simulink model "EMT_load"  (R2024a)
settings: Solver=ode1  StartTime=0.0  StopTime=simtime  FixedStep=Ts  RelTol=1e-3
values from neighbouring files (symbols this model uses):
  c0 = c0_hawk    (= 6.37282e-09)    [EMT_Phasor_parameters.m]
  c1 = c1_hawk    (= 8.76156e-09)    [EMT_Phasor_parameters.m]
  fg = 50    [EMT_Phasor_parameters.m]
  G1gen = 0.1245    [EMT_Phasor_parameters.m]
  G2gen = 0.30    (= 0.3)    [EMT_Phasor_parameters.m]
  G3gen = 0.20    (= 0.2)    [EMT_Phasor_parameters.m]
  G4sgen = 0.2078    [EMT_Phasor_parameters.m]
  G5gen = 0.20    (= 0.2)    [EMT_Phasor_parameters.m]
  G6gen = 0.2078    [EMT_Phasor_parameters.m]
  G6sgen = 0.20    (= 0.2)    [EMT_Phasor_parameters.m]
  G7gen = 0.518    [EMT_Phasor_parameters.m]
  Ihvpk = Ihv*sqrt(2)    [EMT_Phasor_parameters.m]
  l0 = l0_hawk    (= 0.00373)    [EMT_Phasor_parameters.m]
  l1 = l1_hawk    (= 0.00133)    [EMT_Phasor_parameters.m]
  L3dem = 0.10    (= 0.1)    [EMT_Phasor_parameters.m]
  L4dem = 0.30    (= 0.3)    [EMT_Phasor_parameters.m]
  L5dem = 0.35    [EMT_Phasor_parameters.m]
  L6dem = 0.15    [EMT_Phasor_parameters.m]
  L7dem = 0.10    (= 0.1)    [EMT_Phasor_parameters.m]
  Pr = Sr*PF    (= 550050000)    [EMT_Phasor_parameters.m]
  Qr = sqrt(Sr^2 - Pr^2)    [EMT_Phasor_parameters.m]
  r0 = r0_hawk    (= 0.44587)    [EMT_Phasor_parameters.m]
  r1 = r1_hawk    (= 0.12087)    [EMT_Phasor_parameters.m]
  Rtpu = Xtpu/40    (= 0.00375)    [EMT_Phasor_parameters.m]
  S1non = 400e6    (= 400000000)    [EMT_Phasor_parameters.m]
  S2non = 300e6    (= 300000000)    [EMT_Phasor_parameters.m]
  S3non = 200e6    (= 200000000)    [EMT_Phasor_parameters.m]
  S4snon = 200e6    (= 200000000)    [EMT_Phasor_parameters.m]
  S5non = 500e6    (= 500000000)    [EMT_Phasor_parameters.m]
  S6non = 400e6    (= 400000000)    [EMT_Phasor_parameters.m]
  S6snon = 200e6    (= 200000000)    [EMT_Phasor_parameters.m]
  S7non = 200e6    (= 200000000)    [EMT_Phasor_parameters.m]
  simtime = 5    [EMT_Phasor_parameters.m]
  tonvsc = 0.01    [EMT_Phasor_parameters.m]
  Ts = 150e-6    (= 0.00015)    [EMT_Phasor_parameters.m]
  Vhv = 220e3    (= 220000)    [EMT_Phasor_parameters.m]
  Vmv = 22e3    (= 22000)    [EMT_Phasor_parameters.m]
  wc1 = wsw1/10    (= 848.230016469)    [EMT_Phasor_parameters.m]
  wdc1 = wc1/10    (= 84.8230016469)    [EMT_Phasor_parameters.m]
  wpq1 = wc1/10    (= 84.8230016469)    [EMT_Phasor_parameters.m]
  wsw1 = ksw1*2*pi*fg    (= 8482.30016469)    [EMT_Phasor_parameters.m]
  Xtpu = 0.15    [EMT_Phasor_parameters.m]
undefined symbols (not defined in the file or in its folder): D11, Delta, Kf, r, theta0
libraries: simulink_extras x152, spsGroundLib x49, spsCurrentMeasurementLib x39, spsVoltageMeasurementLib x33, simulink x32, eeGeneralControl x32, slpidlib x32, powerlib x30, powerlib_meascontrol x28, spsFirstOrderFilterLib x24, eeTransforms x24, pid_lib x16
(part 16 of 16)

== system EMT_load/G6/VSC/VSC Control/Measurements/EMT/PLL aligned with positive-sequence/Phase-sequence separation ==
  note: Phase-sequence separation based on
      | Delayed Signal Cancellation (DSC) method
  abc : Inport
  Theta : Inport  Port=2
  Complex to Real-Imag1 : ComplexToRealImag
  Complex to Real-Imag2 : ComplexToRealImag
  Complex to Real-Imag3 : ComplexToRealImag
  Constant : Constant  Value=negseq_en
  Demux3 : Demux  Outputs=3
  Exp2 : Math  OutputSignalType=complex
  Exp3 : Math  OutputSignalType=complex
  Gain1 : Gain  Gain=1/2
  Gain4 : Gain  Gain=-1i
  Gain5 : Gain  Gain=1i
  Gain6 : Gain  Gain=1/2
  Gain7 : Gain  Gain=1i
  NOT : Logic  Operator=NOT  IconShape=distinctive  AllPortsSameDT=off  OutDataTypeStr=boolean
  Product3 : Product
  Product4 : Product
  Real-Imag to Complex : RealImagToComplex
  Real-Imag to Complex1 : RealImagToComplex
  Sum1 : Sum  Inputs=|++
  Sum2 : Sum  Inputs=-+|
  Switch : Switch  Criteria=u2 ~= 0  SaturateOnIntegerOverflow=off  InputSameDT=off
  Terminator3 : Terminator
  Transport Delay2 : TransportDelay  DelayTime=1/4*(1/50)
  Transport Delay3 : TransportDelay  DelayTime=1/4*(1/50)
  abc to Alpha-Beta-Zero : spsabctoAlphaBetaZeroLib/abc to Alpha-Beta-Zero
  q+ : Outport
  d+ : Outport  Port=2
  q- : Outport  Port=3
  d- : Outport  Port=4
  wires:
  NOT/1 -> Switch/2
  Constant/1 -> NOT/1
  Switch/1 -> Product3/1
  Gain6/1 -> Switch/3
  Sum2/1 -> Gain1/1
  Transport Delay2/1 -> Real-Imag to Complex1/1
  Demux3/1 -> Real-Imag to Complex/1
  Complex to Real-Imag1/2 -> Transport Delay3/1
  Gain1/1 -> Product4/2
  Real-Imag to Complex/1 -> Complex to Real-Imag1/1, Sum2/2, Sum1/1, Switch/1
  Complex to Real-Imag3/1 -> d-/1
  Real-Imag to Complex1/1 -> Gain5/1
  Complex to Real-Imag1/1 -> Transport Delay2/1
  Transport Delay3/1 -> Real-Imag to Complex1/2
  Demux3/2 -> Real-Imag to Complex/2
  Product3/1 -> Complex to Real-Imag2/1
  Product4/1 -> Complex to Real-Imag3/1
  abc to Alpha-Beta-Zero/1 -> Demux3/1
  abc/1 -> abc to Alpha-Beta-Zero/1
  Exp3/1 -> Product4/1
  Complex to Real-Imag3/2 -> q-/1
  Complex to Real-Imag2/2 -> q+/1
  Demux3/3 -> Terminator3/1
  Sum1/1 -> Gain6/1
  Gain5/1 -> Sum2/1, Sum1/2
  Exp2/1 -> Product3/2
  Gain4/1 -> Exp2/1
  Theta/1 -> Gain4/1, Gain7/1
  Gain7/1 -> Exp3/1
  Complex to Real-Imag2/1 -> d+/1

== system EMT_load/G6/VSC/VSC Control/Measurements/EMT/PLL aligned with positive-sequence/Subsystem ==
  note: PI controller with reset port and initial conditions restored after reset or after maximum/minimum values are reached
  in : Inport
  Reset : Inport  Port=2
  Compare To Constant2 : simulink/Logic and Bit Operations/Compare To Constant  relop=~=  const=0  OutDataTypeStr=boolean
  Constant2 : Constant  Value=2*pi*fg
  Gain : Gain  Gain=kp_pll
  Gain1 : Gain  Gain=kp_pll/tau_pll
  Integrator Limited : Integrator  ExternalReset=level  InitialCondition=2*pi*fg  UpperSaturationLimit=10.1*2*pi*fg  LowerSaturationLimit=0.09*2*pi*fg  ShowSaturationPort=on
  Memory1 : Memory
  NOT : Logic  Operator=NOT  IconShape=distinctive  AllPortsSameDT=off  OutDataTypeStr=boolean
  OR2 : Logic  Operator=OR  IconShape=distinctive  AllPortsSameDT=off  OutDataTypeStr=boolean
  Product : Product
  Sum : Sum
  Switch1 : Switch  SaturateOnIntegerOverflow=off  InputSameDT=off
  w : Outport
  wires:
  Switch1/1 -> w/1
  Product/1 -> Gain1/1, Gain/1
  Gain1/1 -> Integrator Limited/1
  Integrator Limited/2 -> Compare To Constant2/1, Switch1/2
  Compare To Constant2/1 -> Memory1/1
  OR2/1 -> Integrator Limited/2, NOT/1
  Constant2/1 -> Switch1/3
  Memory1/1 -> OR2/1
  Reset/1 -> OR2/2
  Gain/1 -> Sum/1
  Integrator Limited/1 -> Sum/2
  Sum/1 -> Switch1/1
  in/1 -> Product/1
  NOT/1 -> Product/2

== system EMT_load/G6/VSC/VSC Control/Modulation/Phasor I and Phasor PQ/RL time constant/Corrects delay ==
  Clock : Clock
  Gain : Gain  Gain=(2*pi*fg)
  Memory : Memory
  Sum : Sum  Inputs=|+-
  dphi : Outport
  wires:
  Gain/1 -> dphi/1
  Sum/1 -> Gain/1  "Ts"
  Memory/1 -> Sum/2
  Clock/1 -> Sum/1, Memory/1
